simulink model "gmp_pmsm_sensored_nonlinear_sil_mdl_2022b"  (R2022b)
settings: Solver=VariableStepAuto  StartTime=0.0  StopTime=10  RelTol=1e-3
model workspace (MAT data in the model file):
  B = 0
  BW_i = 800
  Flux_t = 0.05895
  IQ24 = Simulink.NumericType
  IQ24.DataTypeMode = 'Fixed-point: binary point scaling'
  IQ24.SignednessBool = 1
  IQ24.WordLength = 32
  IQ24.FixedExponent = -16
  IQ24.SlopeAdjustmentFactor = 1
  IQ24.Bias = 0
  IQ24.DataTypeOverride = 'Inherit'
  IQ24.IsAlias = 0
  IQ24.DataScope = 'Auto'
  J = 0.018
  K_d = 3.72061852168
  K_m = 0.128242020589
  K_u = 0.00236407598332
  Ki_id = 0.001
  Ki_iq = 1
  Ki_n = 25225.1136556
  Kp_id = 1e-05
  Kp_iq = 5e-05
  Kp_n = 12.6125568278
  Ld_t = 0.00303
  Lq_t = 0.02019
  Max_p = 0.006000830667
  P = 2
  RLS_ini_a = 1000000
  Rd_mos = 0.01
  Rs = 0.1215
  Rv = 6.4
  T_final = 0
  T_initial = 0
  Tes = [4 7 10 7 4]
  Tf_t = 0.1
  Tm = 0
  Udq_limit = 550
  Var = 0
  Vce0 = 0
  Vd0 = 0
  Vdc = 80
  button = 1
  im_limit = 40
  mean_prd = 10
  position_init = 0.2
  r_ce = 1e-08
  r_d = 1e-08
  sample_prd = 100
  step_time = 0.2
  ts = 6.25e-05
  wc = 3500
libraries: peripheral_utilities x12, spsSeriesRLCBranchLib x6, spsVoltageMeasurementLib x2, gmp_sil_core_pack x1, spsPermanentMagnetSynchronousMachineLib x1, spsdq0toabcLib x1, spsFourierLib x1, spsControlledVoltageSourceLib x1, spspowerguiLib x1
(part 1 of 2)
settings Model: SimulationMode=accelerator  Creator=javnson  LastModifiedBy=Lin Minyi

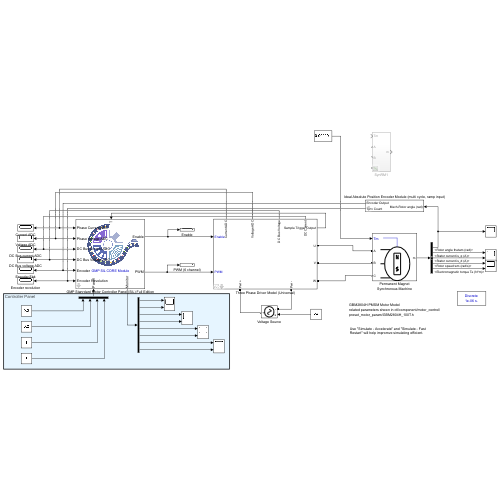
[thumbnail: Simulink's stored preview of the top-level diagram]
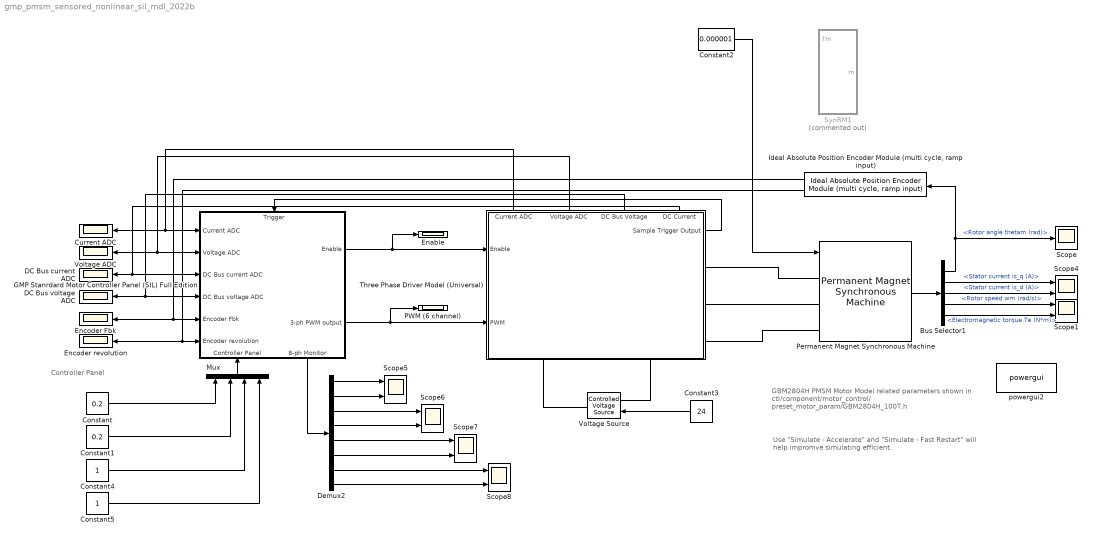
== system gmp_pmsm_sensored_nonlinear_sil_mdl_2022b ==
  note: Use "Simulate - Accelerate" and "Simulate - Fast Restart" will help impromve simulating efficient.
  note: Controller Panel
  note: GBM2804H PMSM Motor Model
      | related parameters shown in ctl/component/motor_control/
      | preset_motor_param/GBM2804H_100T.h
  Bus Selector1 : BusSelector  OutputSignals=Rotor angle thetam (rad),Stator current is_q (A),Stator current is_d (A),Rotor speed wm (rad/s),Electromagnetic torque Te (N*m)
  Constant : Constant  Value=0.2
  Constant1 : Constant  Value=0.2
  Constant2 : Constant  Value=0.000001
  Constant3 : Constant  Value=24
  Constant4 : Constant
  Constant5 : Constant
  Current ADC : Scope
  DC Bus current ADC : Scope
  DC Bus voltage ADC : Scope
  Demux2 : Demux  Outputs=8
  Enable : Scope
  Encoder Fbk : Scope
  Encoder revolution : Scope
  GMP Stanrdard Motor Controller Panel (SIL) Full Edition : Subsystem  mask(GMP SIL Core for single Motor Controller (full edition)){}
      mask help: This is GMP Motor Simulator port.
      settings: PortSchema="{\"entries\":[{\"content\":{\"sides\":[{\"content\":{\"connectorIds\":[\"In1\",\"In2\",\"In3\",\"In4\",\"In5\",\"In6\"]},\"type\":\"ConnectorPlacement.EquallySpacedRectSide\",\"uuid\":\"45c67bc9-9540-469a-a4ac-1e12eb9acca3\"},{\"content\":{\"connectorIds\":[\"Out1\",\"Out2\"],\"side\":\"RIGHT\"},\"type\":\"ConnectorPlacement.EquallySpacedRectSide\",\"uuid\":\"a17116b4-0460-48ab-8ada-a785da6c5e29\"},{\"content\":{\"connectorIds\":[\"In7\"],\"side\":\"TOP\"},\"type\":\"ConnectorPlacement.EquallySpacedRectSide\",\"uuid\":\"15623697-512e-4e4d-ab51-f53c2346fadb\"},{\"content\":{\"connectorIds\":[\"In8\",\"Out3\"],\"side\":\"BOTTOM\"},\"type\":\"ConnectorPlacement.EquallySpacedRectSide\",\"uuid\":\"47f7968c-22c1-4f3d-97d9-242e9dbf8d30\"}]},\"type\":\"ConnectorPlacement.EquallySpacedConnector\",\"uuid\":\"f369880c-e675-4c1f-982e-a4befb03f503\"}],\"packageUris\":[\"http://schema.mathworks.com/mf0/Connector/R2020b\"],\"version\":\"1.0\"}"
      mask DialogControl ParameterGroupVar Prompt: 参数
      mask Display:
      | image(append(fileparts(which('gmp_simulink_utilities.slx')),'\icon\GMP_Core.png'));
      | color('blue');
      | %text(0.3,0.3,'GMP SIL CORE Module','horizontalAlignment','left','verticalAlignment','bottom');
      | disp('\n\n\n\n\n\n\n\nGMP SIL CORE Module');
      | %text(0,0,'y=a*x^2+b','horizontalAlignment','middle', 'verticalAlignment','bottom');
      | 
      | 
      | module_pos = get_param(gcb, 'Position');
      | width = module_pos(3) - module_pos(1);
      | %rectangle('Position',[module_pos(1),module_pos(2),module_pos(3),module_pos(4)],'FaceColor','r');
      | 
      | color('Black');
      | 
      | port_label('output', 1, 'Enable');
      | port_label('output', 2, 'PWM');
      | port_label('output', 3, 'Monitor');
      | 
      | port_label('input', 1, 'Phase Current ADC');
      | port_label('input', 2, 'Phase Voltage ADC');
      | port_label('input', 3, 'DC Bus Current ADC');
      | port_label('input', 4, 'DC Bus Voltage ADC');
      | port_label('input', 5, 'Encoder');
      | port_label('input', 6, 'Encoder Revolution');
      | port_label('input', 7, 'T');
      | port_label('input', 8, 'Panel');
  "Ideal Absolute Position Encoder Module (multi cycle, ramp input)" : peripheral_utilities/Ideal Absolute Position Encoder Module (multi cycle, ramp input)  ENCODER_BIT=14
      settings: SourceProductName=GMP Utilities Library
  Mux : Mux
  PWM (6 channel) : Scope
  Permanent Magnet Synchronous Machine : spsPermanentMagnetSynchronousMachineLib/Permanent Magnet Synchronous Machine  NbPhases=3  FluxDistribution=Sinusoidal  RotorType=Round  MechanicalLoad=Torque Tm  PresetModel=No  ShowDetailedParameters=on  MeasurementBus=off  Resistance=4.7  Inductance=8.5e-3  dqInductances=[8.5e-3,8.5e-3]  La=0.96e-3  MachineConstant=Voltage Constant (V_peak L-L / krpm)  Flux=0.0038197  VoltageCst=1000/206.2  TorqueCst=0.040106  Flat=120  Mechanical=[497e-9 1755e-9 7 0]  PolePairs=4  InitialConditions=[0, 0, 0, 0]  InitialConditions5ph=[0 0 0 0 0 0]  RefAngle=Aligned with phase A axis (original Park)  IterativeDiscreteModel=Trapezoidal non iterative  TsBlock=-1  TsPowergui=0
  Scope : Scope
  Scope{1,4..8} (6 alike) : Scope  NumInputPorts=2
  SynRM1 : Subsystem  Commented=on
  Three Phase Driver Model (Universal) : Subsystem  AncestorBlock=peripheral_utilities/Three Phase Driver Model (Universal)  mask{fswitch=8000, CMP_MAX=6000, Deadband_Upper=48, Deadband_Lower=48, Deadband_us=1, phase_shift=0, R_mosfet_on=0.1, Lon=0, Rd=0.01, Vf=0.3, Rs=1e5, Cs=inf, Rsap=0.005, ADC_GAIN=20, ADC_BIT=12, ADC_REFERENCE=3.3, ADC_BIAS=1.65, ADC_INIT=0, VOLTAGE_ADC_GAIN=0.04049127, VOLTAGE_ADC_BIT=12, VOLTAGE_ADC_REFERENCE=3.3, VOLTAGE_ADC_VOLTAGE=0, VOLTAGE_ADC_INIT=0, VOLTAGE_ADC_CUT_FREQ=1143.4, DCBUS_ADC_GAIN=0.04049127, DCBUS_ADC_BIT=12, DCBUS_ADC_REFERENCE=3.3, DCBUS_ADC_BIAS=0, DCBUS_ADC_INIT=0, DCBUS_CURRENT_ADC_GAIN=1, DCBUS_CURRENT_ADC_BIT=12, DCBUS_CURRENT_ADC_REFERENCE=20, DCBUS_CURRENT_ADC_BIAS=0, DCBUS_CURRENT_ADC_INIT=0}
      mask prompts: DCBUS_CURRENT_ADC_GAIN "DCBUS_ADC_GAIN:"; DCBUS_CURRENT_ADC_BIT "DCBUS_ADC_BIT:"; DCBUS_CURRENT_ADC_REFERENCE "DCBUS_ADC_REFERENCE:"; DCBUS_CURRENT_ADC_BIAS "DCBUS_ADC_BIAS:"; DCBUS_CURRENT_ADC_INIT "DCBUS_ADC_INIT:"
      mask init:
      | calculate_deadband(gcb, 'Deadband_Upper', 'Deadband_Lower',	'CMP_MAX', 'fswitch', 'Deadband_us');
      settings: PortSchema="{\"entries\":[{\"content\":{\"sides\":[{\"content\":{\"connectorIds\":[\"In1\",\"In2\"]},\"type\":\"ConnectorPlacement.EquallySpacedRectSide\",\"uuid\":\"3f4c86ad-0582-4f47-8583-a8af9a7f9adc\"},{\"content\":{\"connectorIds\":[\"Out1\",\"RConn1\",\"RConn2\",\"RConn3\"],\"side\":\"RIGHT\"},\"type\":\"ConnectorPlacement.EquallySpacedRectSide\",\"uuid\":\"ae91f325-3014-4188-9063-296f4d5623fa\"},{\"content\":{\"connectorIds\":[\"Out2\",\"Out3\",\"Out4\",\"Out5\"],\"side\":\"TOP\"},\"type\":\"ConnectorPlacement.EquallySpacedRectSide\",\"uuid\":\"5f2edb36-6849-4a72-b7bd-4d267f120ce4\"},{\"content\":{\"connectorIds\":[\"RConn4\",\"RConn5\"],\"side\":\"BOTTOM\"},\"type\":\"ConnectorPlacement.EquallySpacedRectSide\",\"uuid\":\"79a111ed-6591-4ced-9242-67ea1247c580\"}]},\"type\":\"ConnectorPlacement.EquallySpacedConnector\",\"uuid\":\"8c66eb8e-d25c-472f-a4a5-d1759225ba1c\"}],\"packageUris\":[\"http://schema.mathworks.com/mf0/Connector/R2020b\"],\"version\":\"1.0\"}"
      mask Callback fswitch: calculate_deadband(gcb, 'Deadband_Upper', 'Deadband_Lower',	'CMP_MAX', 'fswitch', 'Deadband_us');
      mask Callback CMP_MAX: calculate_deadband(gcb, 'Deadband_Upper', 'Deadband_Lower',	'CMP_MAX', 'fswitch', 'Deadband_us');
      mask Callback Deadband_Upper: calculate_deadband(gcb, 'Deadband_Upper', 'Deadband_Lower',	'CMP_MAX', 'fswitch', 'Deadband_us');
      mask Callback Deadband_Lower: calculate_deadband(gcb, 'Deadband_Upper', 'Deadband_Lower',	'CMP_MAX', 'fswitch', 'Deadband_us');
      mask DialogControl DescGroupVar Prompt: Three Phases Bridge Peripheral(3-shunt sample)
      mask DialogControl Control21 Prompt: GMP CTL Simulink Utilities: virtual peripherals
      mask DialogControl DescTextVar Prompt: This module provide a ideal 3-phases bridge peripheral.
      mask DialogControl Container4 Prompt: PWM config
      mask DialogControl ParameterGroupVar Prompt: PWM parameters
      mask DialogControl Control2 Prompt: PWM Frequency (Hz):
      mask DialogControl Control4 Prompt: Full Scale PWM Compare value:
      mask DialogControl Control5 Prompt: Deadband Range Set (CMP Value):
      mask DialogControl Control6 Prompt: Deadband time: DEADBAND_CMP/2/CMP_MAX/fswitch
      mask DialogControl Control22 Prompt: Calculated Deadband, us
      mask DialogControl Control20 Prompt: Initial Phase shift:
      mask DialogControl Container5 Prompt: MOSFET config
      mask DialogControl Container7 Prompt: MOSFET parameters
      mask DialogControl Control7 Prompt: Rds(on), unit Ohm
      mask DialogControl Control8 Prompt: Internal diode inducctance, unit H
      mask DialogControl Control9 Prompt: Internal diode resistance Rd, unit Ohm
      mask DialogControl Control10 Prompt: Internal diode forward voltage Vf, unit V
      mask DialogControl Control11 Prompt: Snubber resistance Rs, unit ohm
      mask DialogControl Control12 Prompt: Snubber Capacitance Cs, unit F
      mask DialogControl Container6 Prompt: 3-shunt Current Sample
      mask DialogControl Control13 Prompt: ADC(p.u.) = (real_voltage * ADC_GAIN + ADC_BIAS)/ADC_REFERENCE
      mask DialogControl Control15 Prompt: Shunt Smaple Res, unit Ohm
      mask DialogControl Control14 Prompt: ADC Voltage Gain (Scale Factor):
      mask DialogControl Control16 Prompt: ADC resolution:
      mask DialogControl Control17 Prompt: ADC reference Voltage(V)
      mask DialogControl Control18 Prompt: ADC Bias Voltage(V)
      mask DialogControl Control19 Prompt: ADC Initial Voltage Output (V):
      mask DialogControl Container9 Prompt: 3-shunt Voltage Sample
      mask DialogControl Control34 Prompt: ADC Voltage Gain (Scale Factor):
      mask DialogControl Control23 Prompt: ADC resolution:
      mask DialogControl Control24 Prompt: ADC reference voltage (V), when VOLTAGE_ADC_GAIN = 1, ADC_REF = ADC Full scale
      mask DialogControl Control25 Prompt: ADC Bias Voltage (V):
      mask DialogControl Control26 Prompt: ADC Initial Voltage Output (V):
      mask DialogControl Control27 Prompt: Voltage Filter cut frequency (Hz):
      mask DialogControl Control28 Prompt: Generally, this value less than switch frequency / 10, greater than motor normal frequency * 3
      mask DialogControl Container10 Prompt: DC Bus Voltage Sample
      mask DialogControl Control29 Prompt: ADC Voltage Gain (Scale Factor):
      mask DialogControl Control30 Prompt: ADC resolution:
      mask DialogControl Control32 Prompt: ADC reference voltage (V), when VOLTAGE_ADC_GAIN = 1, ADC_REF = ADC Full scale
      mask DialogControl Control31 Prompt: ADC Bias Voltage (V):
      mask DialogControl Control33 Prompt: ADC Initial Voltage Output (V):
      mask DialogControl Container13 Prompt: DC Bus Current Sample
      mask DialogControl Control29_copy_copy Prompt: ADC Current Gain (Scale Factor):
      mask DialogControl Control30_copy_copy Prompt: ADC resolution:
      mask DialogControl Control32_copy_copy Prompt: ADC reference current (A), when VOLTAGE_ADC_GAIN = 1, ADC_REF = ADC Full scale
      mask DialogControl Control31_copy Prompt: ADC Bias Current (A):
      mask DialogControl Control33_copy Prompt: ADC Initial Current Output (A):
  Voltage ADC : Scope
  Voltage Source : spsControlledVoltageSourceLib/Controlled Voltage Source  Initialize=on  Source_Type=AC  Amplitude=0  Phase=0  Frequency=0  Measurements=None
  powergui2 : spspowerguiLib/powergui  Priority=1  SimulationMode=Discrete  SampleTime=1e-6  frequency=60  Iterations=50  frequencyindice=0  Pbase=100e6  ErrMax=1e-4  UnitsV=kV  UnitsW=MW  buscounter=0  FunctionMessages=off  echomessages=off  EnableUseOfTLC=off  CurrentSourceSwitches=off  DisableSnubberDevices=off  DisableRonSwitches=off  DisableVfSwitches=off  DisplayEquations=off  AutomaticDiscreteSolvers=off  SolverType=Tustin/Backward Euler (TBE)  Interpol=off  ExternalGateDelay=off  methode=off  Ts=100  x0status=blocks  SPID=on  SwTol=0  HookPort=off  NonlinearTolerance=1e-4  nMaxIteration=100  ContinueOnMaxIteration=off  RestoreLinks=warning  ResistiveCurrentMeasurement=off  Frange=[0:2:500]  Ylog=off  Xlog=on  ShowGrid=off  save=off  variable=ZData  structure=0  ZoomFFT=off  StartTime=0.0  cycles=1  DisplayStyle=1  fundamental=60  FreqAxis=off  MaxFrequency=1000  frequencyindicesteady=1  RmsSteady=1  display=off
  wires:
  GMP Stanrdard Motor Controller Panel (SIL) Full Edition/1(Enable) -> Three Phase Driver Model (Universal)/1(Enable), Enable/1
  GMP Stanrdard Motor Controller Panel (SIL) Full Edition/2(3-ph PWM output) -> PWM (6 channel)/1, Three Phase Driver Model (Universal)/2(PWM)
  Constant2/1 -> Permanent Magnet Synchronous Machine/1
  Three Phase Driver Model (Universal)/1(Sample Trigger Output) -> GMP Stanrdard Motor Controller Panel (SIL) Full Edition/7(Trigger)
  Three Phase Driver Model (Universal)/2(Current ADC) -> GMP Stanrdard Motor Controller Panel (SIL) Full Edition/1(Current ADC), Current ADC/1
  Three Phase Driver Model (Universal)/3(Voltage ADC) -> GMP Stanrdard Motor Controller Panel (SIL) Full Edition/2(Voltage ADC), Voltage ADC/1
  Three Phase Driver Model (Universal)/4(DC Bus Voltage) -> DC Bus voltage ADC/1, GMP Stanrdard Motor Controller Panel (SIL) Full Edition/4(DC Bus voltage ADC)
  Permanent Magnet Synchronous Machine/1 -> Bus Selector1/1
  Bus Selector1/1 -> "Ideal Absolute Position Encoder Module (multi cycle, ramp input)"/1, Scope/1  "<Rotor angle thetam (rad)>"
  "Ideal Absolute Position Encoder Module (multi cycle, ramp input)"/1 -> Encoder Fbk/1, GMP Stanrdard Motor Controller Panel (SIL) Full Edition/5(Encoder Fbk)
  Bus Selector1/3 -> Scope4/2  "<Stator current is_d (A)>"
  Bus Selector1/2 -> Scope4/1  "<Stator current is_q (A)>"
  Constant3/1 -> Voltage Source/1
  Demux2/4 -> Scope6/2
  Demux2/3 -> Scope6/1
  Demux2/2 -> Scope5/2
  Demux2/1 -> Scope5/1
  GMP Stanrdard Motor Controller Panel (SIL) Full Edition/3(8-ph Monitor) -> Demux2/1
  Bus Selector1/4 -> Scope1/1  "<Rotor speed wm (rad/s)>"
  Bus Selector1/5 -> Scope1/2  "<Electromagnetic torque Te (N*m)>"
  "Ideal Absolute Position Encoder Module (multi cycle, ramp input)"/2 -> Encoder revolution/1, GMP Stanrdard Motor Controller Panel (SIL) Full Edition/6(Encoder revolution)
  Mux/1 -> GMP Stanrdard Motor Controller Panel (SIL) Full Edition/8(Controller Panel)
  Constant/1 -> Mux/1
  Constant1/1 -> Mux/2
  Constant4/1 -> Mux/3
  Constant5/1 -> Mux/4
  Demux2/5 -> Scope7/1
  Demux2/6 -> Scope7/2
  Demux2/7 -> Scope8/1
  Demux2/8 -> Scope8/2
  Three Phase Driver Model (Universal)/5(DC Current) -> DC Bus current ADC/1, GMP Stanrdard Motor Controller Panel (SIL) Full Edition/3(DC Bus current ADC)
  connections:
  Permanent Magnet Synchronous Machine/LConn2 -- Three Phase Driver Model (Universal)/RConn2
  Permanent Magnet Synchronous Machine/LConn3 -- Three Phase Driver Model (Universal)/RConn3
  Permanent Magnet Synchronous Machine/LConn1 -- Three Phase Driver Model (Universal)/RConn1
  Three Phase Driver Model (Universal)/RConn5 -- Voltage Source/LConn1
  Three Phase Driver Model (Universal)/RConn4 -- Voltage Source/RConn1

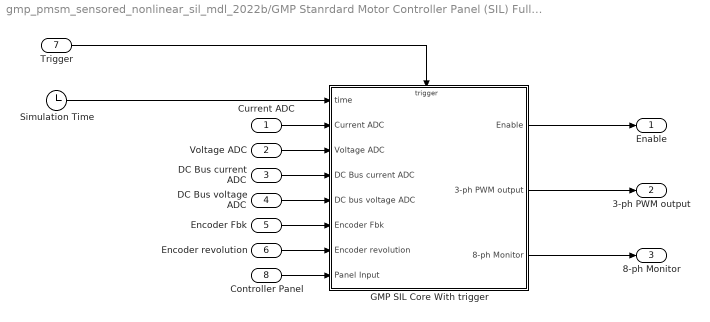
== system gmp_pmsm_sensored_nonlinear_sil_mdl_2022b/GMP Stanrdard Motor Controller Panel (SIL) Full Edition ==
  Current ADC : Inport
  Voltage ADC : Inport  Port=2
  DC Bus current ADC : Inport  Port=3
  DC Bus voltage ADC : Inport  Port=4
  Encoder Fbk : Inport  Port=5
  Encoder revolution : Inport  Port=6
  Trigger : Inport  Port=7
  Controller Panel : Inport  Port=8
  GMP SIL Core With trigger : Subsystem
  Simulation Time : Clock
  Enable : Outport
  3-ph PWM output : Outport  Port=2
  8-ph Monitor : Outport  Port=3
  wires:
  Encoder Fbk/1 -> GMP SIL Core With trigger/6(Encoder Fbk)
  Encoder revolution/1 -> GMP SIL Core With trigger/7(Encoder revolution)
  GMP SIL Core With trigger/2(3-ph PWM output) -> 3-ph PWM output/1
  Simulation Time/1 -> GMP SIL Core With trigger/1(time)
  GMP SIL Core With trigger/1(Enable) -> Enable/1
  Voltage ADC/1 -> GMP SIL Core With trigger/3(Voltage ADC)
  Current ADC/1 -> GMP SIL Core With trigger/2(Current ADC)
  GMP SIL Core With trigger/3(8-ph Monitor) -> 8-ph Monitor/1
  DC Bus current ADC/1 -> GMP SIL Core With trigger/4(DC Bus current ADC)
  Trigger/1 -> GMP SIL Core With trigger/Trigger
  DC Bus voltage ADC/1 -> GMP SIL Core With trigger/5(DC bus voltage ADC)
  Controller Panel/1 -> GMP SIL Core With trigger/8(Panel Input)

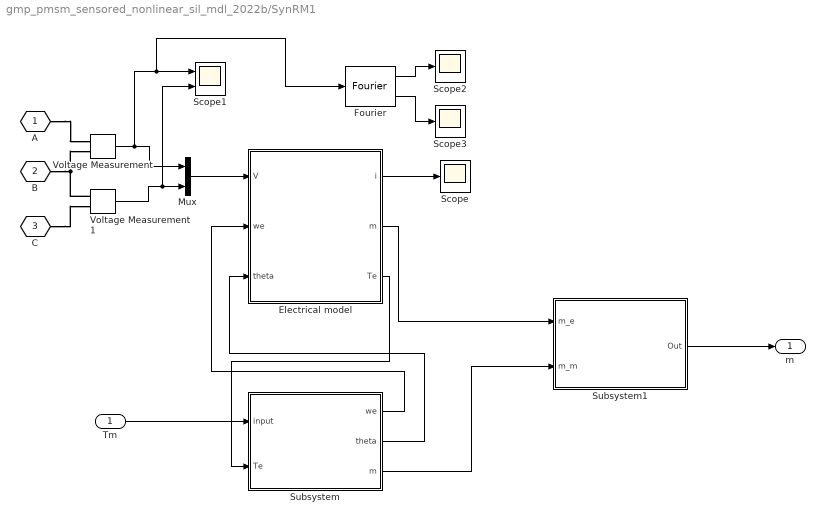
== system gmp_pmsm_sensored_nonlinear_sil_mdl_2022b/SynRM1 ==
  Tm : Inport
  Electrical model : Subsystem
  Fourier : spsFourierLib/Fourier  Freq=100  n=1  InInit=[0, 0]  Ts=0
  Mux : Mux  Inputs=2
  Scope : Scope
  Scope1 : Scope  NumInputPorts=2
  Scope2 : Scope
  Scope3 : Scope
  Subsystem : Subsystem
  Subsystem1 : Subsystem
  Voltage Measurement : spsVoltageMeasurementLib/Voltage Measurement  PhasorSimulation=off  OutputType=Complex  PSBequivalent=0
  Voltage Measurement1 : spsVoltageMeasurementLib/Voltage Measurement  PhasorSimulation=off  OutputType=Complex  PSBequivalent=0
  A : PMIOPort  Side=Left
  B : PMIOPort  Port=2  Side=Left
  C : PMIOPort  Port=3  Side=Left
  m : Outport  VectorParamsAs1DForOutWhenUnconnected=off
  wires:
  Subsystem/3(m) -> Subsystem1/2(m_m)
  Subsystem/1(we) -> Electrical model/2(we)
  Mux/1 -> Electrical model/1(V)
  Subsystem/2(theta) -> Electrical model/3(theta)
  Electrical model/3(Te) -> Subsystem/2(Te)
  Subsystem1/1(Out) -> m/1
  Electrical model/1(i) -> Scope/1
  Electrical model/2(m) -> Subsystem1/1(m_e)
  Tm/1 -> Subsystem/1(input)
  Voltage Measurement/1 -> Fourier/1, Scope1/1, Mux/1
  Voltage Measurement1/1 -> Scope1/2, Mux/2
  Fourier/1 -> Scope2/1
  Fourier/2 -> Scope3/1
  connections:
  C/RConn1 -- Voltage Measurement1/LConn2
  A/RConn1 -- Voltage Measurement/LConn1
  B/RConn1 -- Voltage Measurement1/LConn1 -- Voltage Measurement/LConn2

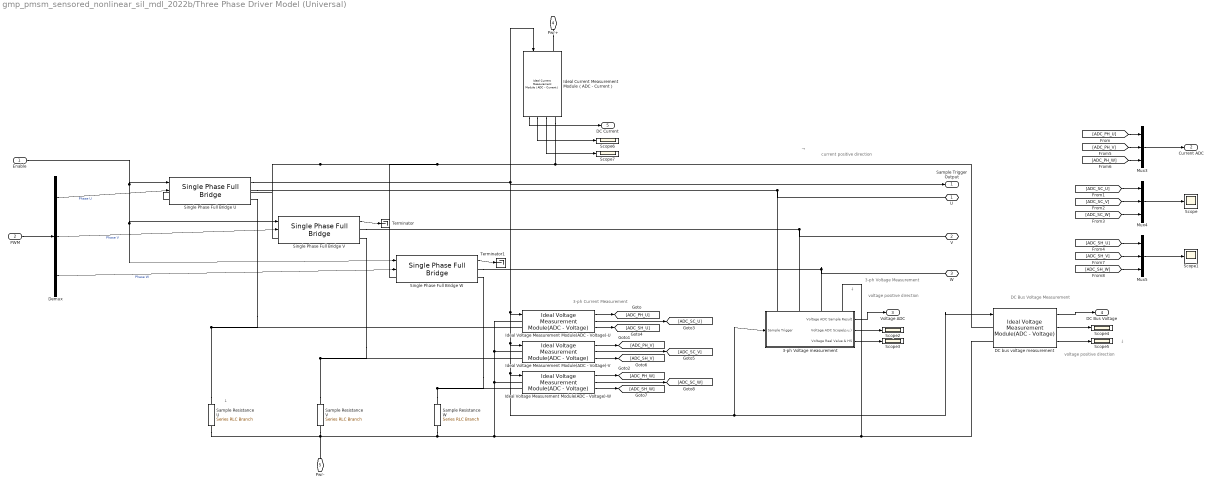
== system gmp_pmsm_sensored_nonlinear_sil_mdl_2022b/Three Phase Driver Model (Universal) ==
  note: 3-ph Current Measurement
  note: →
  note: current positive direction
  note: ↓
  note: voltage positive direction
  note: ↓
  note: 3-ph Voltage Measurement
  note: DC Bus Voltage Measurement
  note: ↓
  note: voltage positive direction
  Enable : Inport
  PWM : Inport  Port=2
  3-ph Voltage measurement : Subsystem  AncestorBlock=peripheral_utilities/Three Phases Voltage (ph-gnd) Measurement with Filter  mask{ADC_GAIN=VOLTAGE_ADC_GAIN, ADC_BIT=VOLTAGE_ADC_BIT, ADC_REFERENCE=VOLTAGE_ADC_REFERENCE, ADC_BIAS=VOLTAGE_ADC_VOLTAGE, ADC_INIT=VOLTAGE_ADC_INIT, cut_frequency=VOLTAGE_ADC_CUT_FREQ}
      settings: PortSchema="{\"entries\":[{\"content\":{\"sides\":[{\"content\":{\"connectorIds\":[\"In1\"]},\"type\":\"ConnectorPlacement.EquallySpacedRectSide\",\"uuid\":\"ae4f4612-c092-4fa0-8a43-5c9e823110e3\"},{\"content\":{\"connectorIds\":[\"Out1\",\"Out2\",\"Out3\"],\"side\":\"RIGHT\"},\"type\":\"ConnectorPlacement.EquallySpacedRectSide\",\"uuid\":\"6db15ef0-d33a-4775-b4e6-14a566796673\"},{\"content\":{\"connectorIds\":[\"LConn1\",\"LConn2\",\"LConn3\",\"LConn4\"],\"side\":\"TOP\"},\"type\":\"ConnectorPlacement.EquallySpacedRectSide\",\"uuid\":\"cfddd664-59f3-497b-b33e-fe832fe7a7bd\"}]},\"type\":\"ConnectorPlacement.EquallySpacedConnector\",\"uuid\":\"5bacf0ad-0c4a-4f47-a242-d8a476ab7f52\"}],\"packageUris\":[\"http://schema.mathworks.com/mf0/Connector/R2020b\"],\"version\":\"1.0\"}"
      mask DialogControl DescGroupVar Prompt: 3 phases Voltage Sample ADC Model
      mask DialogControl Control10 Prompt: GMP CTL Simulink Utilities: virtual peripherals
      mask DialogControl DescTextVar Prompt: This is a ideal Voltage Measurement Module.
      mask DialogControl Control2 Prompt: ADC(p.u.) = (real_voltage * ADC_GAIN + ADC_BIAS)/ADC_REFERENCE
      mask DialogControl ParameterGroupVar Prompt: parameters:
      mask DialogControl Control3 Prompt: ADC Voltage Gain (Scale Factor):
      mask DialogControl Control4 Prompt: ADC resolution:
      mask DialogControl Control5 Prompt: ADC reference Voltage (V), when ADC_GAIN=1, ADC_REF = ADC full scale
      mask DialogControl Control6 Prompt: ADC Bias Voltage(V)
      mask DialogControl Control7 Prompt: ADC Initial Voltage Output (V):
      mask DialogControl Control8 Prompt: Voltage Filter cut frequency (Hz):
      mask DialogControl Control9 Prompt: Generally, this value less than switch frequency / 10, greater than motor normal frequency * 3
  DC bus voltage measurement : peripheral_utilities/Ideal Voltage Measurement Module(ADC - Voltage)  ADC_GAIN=DCBUS_ADC_GAIN  ADC_BIT=DCBUS_ADC_BIT  ADC_REFERENCE=DCBUS_ADC_REFERENCE  ADC_BIAS=DCBUS_ADC_BIAS  ADC_INIT=DCBUS_ADC_INIT
      settings: SourceProductName=GMP Utilities Library
  Demux : Demux  Outputs=3
  Ideal Current Measurement Module（ADC - Current） : peripheral_utilities/Ideal Current Measurement Module（ADC - Current）  ADC_GAIN=DCBUS_CURRENT_ADC_GAIN  ADC_BIT=DCBUS_CURRENT_ADC_BIT  ADC_REFERENCE=DCBUS_CURRENT_ADC_REFERENCE  ADC_BIAS=DCBUS_CURRENT_ADC_BIAS  ADC_INIT=DCBUS_CURRENT_ADC_INIT
      settings: SourceProductName=GMP Utilities Library
  Ideal Voltage Measurement Module(ADC - Voltage)-U : peripheral_utilities/Ideal Voltage Measurement Module(ADC - Voltage)  ADC_GAIN=ADC_GAIN  ADC_BIT=ADC_BIT  ADC_REFERENCE=ADC_REFERENCE  ADC_BIAS=ADC_BIAS  ADC_INIT=ADC_INIT
      settings: SourceProductName=GMP Utilities Library
  Ideal Voltage Measurement Module(ADC - Voltage)-V : peripheral_utilities/Ideal Voltage Measurement Module(ADC - Voltage)  ADC_GAIN=ADC_GAIN  ADC_BIT=ADC_BIT  ADC_REFERENCE=ADC_REFERENCE  ADC_BIAS=ADC_BIAS  ADC_INIT=ADC_INIT
      settings: SourceProductName=GMP Utilities Library
  Ideal Voltage Measurement Module(ADC - Voltage)-W : peripheral_utilities/Ideal Voltage Measurement Module(ADC - Voltage)  ADC_GAIN=ADC_GAIN  ADC_BIT=ADC_BIT  ADC_REFERENCE=ADC_REFERENCE  ADC_BIAS=ADC_BIAS  ADC_INIT=ADC_INIT
      settings: SourceProductName=GMP Utilities Library
  Mux3 : Mux  Inputs=3
  Mux4 : Mux  Inputs=3
  Mux5 : Mux  Inputs=3
  Sample Resistance U : spsSeriesRLCBranchLib/Series RLC Branch  LConnTagsString=__new0  RConnTagsString=__new0  BranchType=R  Resistance=Rsap  Inductance=1e-3  SetiL0=off  InitialCurrent=0  Capacitance=1e-6  Setx0=off  InitialVoltage=0  Measurements=None
  Sample Resistance V : spsSeriesRLCBranchLib/Series RLC Branch  LConnTagsString=__new0  RConnTagsString=__new0  BranchType=R  Resistance=Rsap  Inductance=1e-3  SetiL0=off  InitialCurrent=0  Capacitance=1e-6  Setx0=off  InitialVoltage=0  Measurements=None
  Sample Resistance W : spsSeriesRLCBranchLib/Series RLC Branch  LConnTagsString=__new0  RConnTagsString=__new0  BranchType=R  Resistance=Rsap  Inductance=1e-3  SetiL0=off  InitialCurrent=0  Capacitance=1e-6  Setx0=off  InitialVoltage=0  Measurements=None
  Scope{,1..7} (8 alike) : Scope
  Single Phase Full Bridge U : peripheral_utilities/Single Phase Full Bridge  fswitch=fswitch  CMP_MAX=CMP_MAX  Deadband_Upper=Deadband_Upper  Deadband_Lower=Deadband_Lower  Deadband_us=NaN  phase_shift=phase_shift  R_mosfet_on=R_mosfet_on  Lon=Lon  Rd=Rd  Vf=Vf  Rs=Rs  Cs=Cs
      settings: SourceProductName=GMP Utilities Library
  Single Phase Full Bridge V : peripheral_utilities/Single Phase Full Bridge  fswitch=fswitch  CMP_MAX=CMP_MAX  Deadband_Upper=Deadband_Upper  Deadband_Lower=Deadband_Lower  Deadband_us=NaN  phase_shift=phase_shift  R_mosfet_on=R_mosfet_on  Lon=Lon  Rd=Rd  Vf=Vf  Rs=Rs  Cs=Cs
      settings: SourceProductName=GMP Utilities Library
  Single Phase Full Bridge W : peripheral_utilities/Single Phase Full Bridge  fswitch=fswitch  CMP_MAX=CMP_MAX  Deadband_Upper=Deadband_Upper  Deadband_Lower=Deadband_Lower  Deadband_us=NaN  phase_shift=phase_shift  R_mosfet_on=R_mosfet_on  Lon=Lon  Rd=Rd  Vf=Vf  Rs=Rs  Cs=Cs
      settings: SourceProductName=GMP Utilities Library
  Terminator : Terminator
  Terminator1 : Terminator
  U : PMIOPort  Side=Right
  V : PMIOPort  Port=2  Side=Right
  W : PMIOPort  Port=3  Side=Right
  Pwr+ : PMIOPort  Port=4  Side=Right
  Pwr- : PMIOPort  Port=5  Side=Right
  Sample Trigger Output : Outport
  Current ADC : Outport  Port=2
  Voltage ADC : Outport  Port=3
  DC Bus Voltage : Outport  Port=4
  DC Current : Outport  Port=5
  wires:
  Demux/1 -> Single Phase Full Bridge U/2  "Phase U"
  Ideal Voltage Measurement Module(ADC - Voltage)-U/1 -> [ADC_PH_U]
  Single Phase Full Bridge V/1 -> Terminator/1
  Single Phase Full Bridge W/1 -> Terminator1/1
  Ideal Voltage Measurement Module(ADC - Voltage)-U/2 -> [ADC_SC_U]
  Demux/2 -> Single Phase Full Bridge V/2  "Phase V"
  Demux/3 -> Single Phase Full Bridge W/2  "Phase W"
  [ADC_PH_V] -> Mux3/2
  [ADC_SC_V] -> Mux4/2
  Ideal Voltage Measurement Module(ADC - Voltage)-U/3 -> [ADC_SH_U]
  Mux3/1 -> Current ADC/1
  Ideal Voltage Measurement Module(ADC - Voltage)-V/1 -> [ADC_PH_V]
  [ADC_SC_U] -> Mux4/1
  [ADC_SH_W] -> Mux5/3
  Mux5/1 -> Scope1/1
  Ideal Voltage Measurement Module(ADC - Voltage)-W/1 -> [ADC_PH_W]
  [ADC_PH_U] -> Mux3/1
  Enable/1 -> Single Phase Full Bridge V/1, Single Phase Full Bridge W/1, Single Phase Full Bridge U/1
  Mux4/1 -> Scope/1
  Ideal Voltage Measurement Module(ADC - Voltage)-V/3 -> [ADC_SH_V]
  Single Phase Full Bridge U/1 -> Sample Trigger Output/1, Ideal Current Measurement Module（ADC - Current）/1, Ideal Voltage Measurement Module(ADC - Voltage)-V/1, Ideal Voltage Measurement Module(ADC - Voltage)-W/1, DC bus voltage measurement/1, 3-ph Voltage measurement/1(Sample Trigger), Ideal Voltage Measurement Module(ADC - Voltage)-U/1
  [ADC_SH_U] -> Mux5/1
  Ideal Voltage Measurement Module(ADC - Voltage)-V/2 -> [ADC_SC_V]
  Ideal Voltage Measurement Module(ADC - Voltage)-W/3 -> [ADC_SH_W]
  [ADC_PH_W] -> Mux3/3
  [ADC_SC_W] -> Mux4/3
  [ADC_SH_V] -> Mux5/2
  Ideal Voltage Measurement Module(ADC - Voltage)-W/2 -> [ADC_SC_W]
  3-ph Voltage measurement/1(Voltage ADC Sample Result) -> Voltage ADC/1
  3-ph Voltage measurement/2(Voltage ADC Scope(p.u.)) -> Scope2/1
  3-ph Voltage measurement/3(Voltage Real Value & HS) -> Scope3/1
  DC bus voltage measurement/1 -> DC Bus Voltage/1
  DC bus voltage measurement/2 -> Scope4/1
  DC bus voltage measurement/3 -> Scope5/1
  PWM/1 -> Demux/1
  Ideal Current Measurement Module（ADC - Current）/1 -> DC Current/1
  Ideal Current Measurement Module（ADC - Current）/2 -> Scope6/1
  Ideal Current Measurement Module（ADC - Current）/3 -> Scope7/1
  connections:
  Single Phase Full Bridge V/RConn1 -- V/RConn1 -- 3-ph Voltage measurement/LConn2
  Single Phase Full Bridge U/RConn1 -- U/RConn1 -- 3-ph Voltage measurement/LConn1
  Single Phase Full Bridge W/RConn1 -- W/RConn1 -- 3-ph Voltage measurement/LConn3
  Sample Resistance V/LConn1 -- Ideal Voltage Measurement Module(ADC - Voltage)-V/LConn2 -- Single Phase Full Bridge V/RConn2
  Pwr-/RConn1 -- Sample Resistance U/RConn1 -- Sample Resistance V/RConn1 -- Sample Resistance W/RConn1 -- 3-ph Voltage measurement/LConn4 -- DC bus voltage measurement/LConn2 -- Ideal Voltage Measurement Module(ADC - Voltage)-U/LConn1 -- Ideal Voltage Measurement Module(ADC - Voltage)-V/LConn1 -- Ideal Voltage Measurement Module(ADC - Voltage)-W/LConn1
  Sample Resistance W/LConn1 -- Ideal Voltage Measurement Module(ADC - Voltage)-W/LConn2 -- Single Phase Full Bridge W/RConn2
  Sample Resistance U/LConn1 -- Ideal Voltage Measurement Module(ADC - Voltage)-U/LConn2 -- Single Phase Full Bridge U/RConn2
  DC bus voltage measurement/LConn1 -- Ideal Current Measurement Module（ADC - Current）/RConn1 -- Single Phase Full Bridge W/LConn1 -- Single Phase Full Bridge U/LConn1 -- Single Phase Full Bridge V/LConn1
  Pwr+/RConn1 -- Ideal Current Measurement Module（ADC - Current）/LConn1

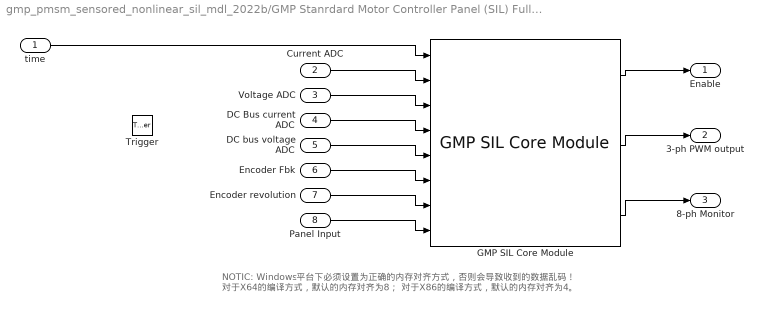
== system gmp_pmsm_sensored_nonlinear_sil_mdl_2022b/GMP Stanrdard Motor Controller Panel (SIL) Full Edition/GMP SIL Core With trigger ==
  note: NOTIC:
      | Windows平台下必须设置为正确的内存对齐方式，否则会导致收到的数据乱码！
      | 对于X64的编译方式，默认的内存对齐为8；
      | 对于X86的编译方式，默认的内存对齐为4。
  time : Inport
  Current ADC : Inport  Port=2
  Voltage ADC : Inport  Port=3
  DC Bus current ADC : Inport  Port=4
  DC bus voltage ADC : Inport  Port=5
  Encoder Fbk : Inport  Port=6
  Encoder revolution : Inport  Port=7
  Panel Input : Inport  Port=8
  Trigger : TriggerPort  VariantControl=(inherit)  PortDimensions=1
  GMP SIL Core Module : gmp_sil_core_pack/GMP SIL Core Module  MaskPackedDataTypes={'double','uint32','uint32','uint32','uint32', 'uint32', 'int32', 'double'}  MaskPackedDataSizes={[1],[3],[3],[1],[1], [1], [1], [4]}  MaskUnpackedDataTypes={'double', 'uint32','double'}  MaskUnpackedDataSizes={[1],[3],[8]}  MaskAlignment=1  MaskHostAddr='127.0.0.1'  MaskMsgTxPort=12300  MaskMsgRxPort=12301  MaskCmdTxPort=12302  MaskCmdRxPort=12303
      settings: SourceProductName=GMP Utilities Library
  Enable : Outport
  3-ph PWM output : Outport  Port=2
  8-ph Monitor : Outport  Port=3
  wires:
  Current ADC/1 -> GMP SIL Core Module/2
  Voltage ADC/1 -> GMP SIL Core Module/3
  DC Bus current ADC/1 -> GMP SIL Core Module/4
  time/1 -> GMP SIL Core Module/1
  GMP SIL Core Module/3 -> 8-ph Monitor/1
  GMP SIL Core Module/2 -> 3-ph PWM output/1
  GMP SIL Core Module/1 -> Enable/1
  Encoder Fbk/1 -> GMP SIL Core Module/6
  Encoder revolution/1 -> GMP SIL Core Module/7
  DC bus voltage ADC/1 -> GMP SIL Core Module/5
  Panel Input/1 -> GMP SIL Core Module/8

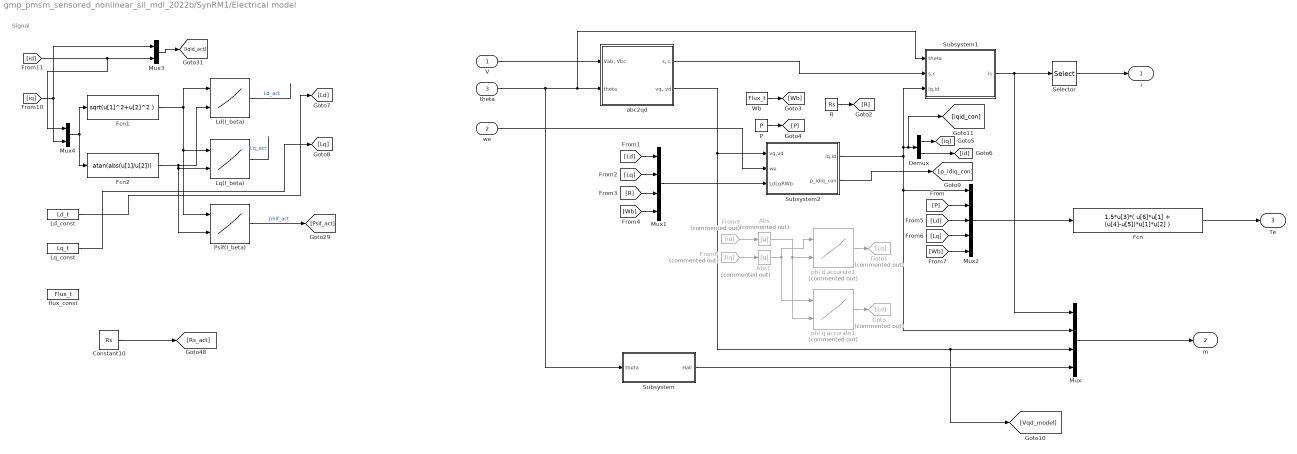
== system gmp_pmsm_sensored_nonlinear_sil_mdl_2022b/SynRM1/Electrical model ==
  note: Signal
  V : Inport
  we : Inport  Port=2
  theta : Inport  Port=3
  Abs : Abs  Commented=on  SaturateOnIntegerOverflow=off
  Abs1 : Abs  Commented=on  SaturateOnIntegerOverflow=off
  Constant10 : Constant  Value=Rs
  Demux : Demux  Outputs=2
  Fcn : Fcn  Expr=1.5*u[3]*( u[6]*u[1] + (u[4]-u[5])*u[1]*u[2] )
  Fcn1 : Fcn  Expr=sqrt(u[1]^2+u[2]^2 )
  Fcn2 : Fcn  Expr=atan(abs(u[1]/u[2]))
  From8 : From  Commented=on  GotoTag=iq
  From9 : From  Commented=on  GotoTag=id
  Goto : Goto  Commented=on  GotoTag=Ld
  Goto1 : Goto  Commented=on  GotoTag=Lq
  Ld(I_beta) : Lookup_n-D  BreakpointsForDimension1=[0,4,8,12,16,20,24,28,32,36,40,44,48,52,56,60,64,68,72,76]  BreakpointsForDimension2=[0,4,8,12,16,20,24,28,32,36,40,44,48,52,56,60,64,68,72,76,80,84,88,90]  Table=[0.0090049,0.0090049,0.0090049,0.0090049,0.0090049,0.0090049,0.0090049,0.0090049,0.0090049,0.0090049,0.0090049,0.0090049,0.0090049,0.0090049,0.0090049,0.0090049,0.0090049,0.0090049,0.0090049,0.0090049,0.0090049,0.0090049,0.0090049,0.0090049;0.0091068,0.0083359,0.0077182,0.0071952,0.0067602,0.0063986,0.0061075,0.0058615,0.0056442,0.0054621,0.0053073,0.0051722,0.0050586,0.0049576,0.0048709,0.0047948,0.0047272,0.0046738,0.0046308,0.0045967,0.00457,0.0045527,0.0045425,0.0045403;0.0093464,0.0079938,0.0070425,0.006355,0.0058504,0.0054685,0.005168,0.004922,0.0047173,0.0045442,0.0044053,0.0042808,0.0041752,0.0040816,0.0040014,0.0039315,0.0038713,0.0038189,0.0037747,0.0037414,0.0037159,0.0036999,0.0036913,0.0036904;0.0094184,0.0086648,0.007532,0.0065799,0.0059032,0.0053778,0.0049522,0.0046235,0.0043749,0.0041848,0.0040338,0.0039102,0.0038062,0.0037163,0.0036343,0.0035659,0.003505,0.0034522,0.0034077,0.003372,0.0033446,0.0033271,0.0033182,0.003317;0.007537,0.0073523,0.0068251,0.0060935,0.0054955,0.0050421,0.0046797,0.0043924,0.0041627,0.0039813,0.0038382,0.003715,0.0036051,0.0035122,0.0034334,0.0033641,0.0033014,0.0032455,0.0031985,0.00316,0.0031309,0.0031118,0.0031022,0.0031011;0.0069136,0.0066119,0.0061429,0.0055601,0.0050595,0.0046689,0.004363,0.0041106,0.0039094,0.0037548,0.0036311,0.0035297,0.003445,0.0033686,0.0032942,0.0032267,0.0031671,0.0031114,0.0030613,0.0030204,0.0029894,0.002969,0.0029587,0.0029574;0.0067888,0.0062678,0.005688,0.0051372,0.0047121,0.0043706,0.0040971,0.0038745,0.0037001,0.0035638,0.0034559,0.0033682,0.0032948,0.0032327,0.0031761,0.0031194,0.0030631,0.0030118,0.0029628,0.0029201,0.0028873,0.0028657,0.002855,0.0028536;0.0064852,0.0059179,0.0053416,0.0048215,0.0044208,0.0041168,0.0038718,0.0036757,0.0035267,0.0034084,0.0033126,0.0032335,0.0031693,0.0031162,0.0030692,0.0030242,0.0029766,0.0029286,0.0028841,0.0028423,0.0028087,0.0027864,0.0027753,0.0027739;0.0061523,0.0056113,0.0050565,0.0045719,0.0041984,0.0039199,0.0036926,0.0035158,0.0033808,0.0032752,0.0031919,0.0031227,0.0030647,0.0030165,0.0029765,0.0029393,0.0029008,0.0028583,0.002817,0.002778,0.0027453,0.0027227,0.0027115,0.0027103;0.0058954,0.0053596,0.0048097,0.0043561,0.0040148,0.0037503,0.0035417,0.0033833,0.0032591,0.0031631,0.0030877,0.0030266,0.0029757,0.0029326,0.0028962,0.0028645,0.0028327,0.0027967,0.0027584,0.0027223,0.002691,0.0026694,0.0026587,0.0026572;0.0056976,0.0051489,0.0045961,0.004167,0.0038525,0.0036066,0.0034122,0.0032677,0.0031545,0.0030661,0.0029972,0.0029426,0.0028976,0.0028598,0.0028271,0.0027991,0.0027724,0.0027421,0.002707,0.0026731,0.0026436,0.0026234,0.0026135,0.0026121;0.0055231,0.0049627,0.0044187,0.0040007,0.0037069,0.0034785,0.0032983,0.0031643,0.0030617,0.0029804,0.0029182,0.0028686,0.0028288,0.0027956,0.0027666,0.0027417,0.0027187,0.0026929,0.0026618,0.0026296,0.0026011,0.0025825,0.0025738,0.0025727;0.0053694,0.0047911,0.0042535,0.0038565,0.0035785,0.0033645,0.0031988,0.0030752,0.0029797,0.0029055,0.0028481,0.0028031,0.002767,0.0027377,0.002713,0.0026907,0.0026708,0.0026487,0.0026213,0.0025909,0.0025632,0.0025454,0.0025381,0.0025373;0.0052237,0.0046319,0.0041064,0.0037302,0.0034662,0.0032628,0.0031101,0.0029956,0.0029078,0.0028387,0.0027859,0.0027449,0.0027117,0.0026861,0.0026645,0.0026452,0.0026275,0.0026087,0.0025847,0.002556,0.0025292,0.0025117,0.0025053,0.0025047;0.0050914,0.0044851,0.003973,0.0036151,0.0033625,0.0031734,0.0030322,0.0029247,0.0028431,0.0027797,0.0027305,0.0026924,0.0026625,0.0026388,0.0026201,0.002604,0.0025886,0.0025725,0.0025511,0.0025243,0.0024983,0.0024809,0.0024746,0.0024742;0.004977,0.004351,0.0038492,0.0035074,0.0032708,0.0030953,0.0029629,0.0028607,0.0027852,0.0027265,0.002681,0.0026455,0.0026177,0.0025961,0.0025796,0.0025663,0.0025528,0.0025391,0.0025203,0.0024953,0.00247,0.0024526,0.002446,0.0024453;0.0048627,0.0042246,0.0037365,0.0034117,0.0031881,0.0030249,0.0028998,0.002804,0.0027327,0.0026783,0.0026359,0.0026029,0.0025771,0.0025573,0.0025427,0.0025312,0.0025199,0.0025084,0.0024918 ...(+761 chars)]  InterpMethod=Akima spline  RndMeth=Simplest
      settings: InputPortMap=u0,u1
  Ld_const : Constant  Value=Ld_t
  Lq(I_beta) : Lookup_n-D  BreakpointsForDimension1=[0,4,8,12,16,20,24,28,32,36,40,44,48,52,56,60,64,68,72,76]  BreakpointsForDimension2=[0,4,8,12,16,20,24,28,32,36,40,44,48,52,56,60,64,68,72,76,80,84,88,90]  Table=[0.027272,0.027272,0.027272,0.027272,0.027272,0.027272,0.027272,0.027272,0.027272,0.027272,0.027272,0.027272,0.027272,0.027272,0.027272,0.027272,0.027272,0.027272,0.027272,0.027272,0.027272,0.027272,0.027272,0.027272;0.027457,0.027451,0.027443,0.027434,0.027425,0.027414,0.027402,0.02739,0.027376,0.027361,0.027345,0.027328,0.027312,0.027294,0.027277,0.02726,0.027243,0.027228,0.027214,0.027202,0.027193,0.027187,0.027183,0.027183;0.027424,0.02742,0.027429,0.027443,0.027463,0.027488,0.027502,0.027506,0.027502,0.027489,0.02747,0.027448,0.02742,0.027389,0.027353,0.027315,0.027274,0.027232,0.02719,0.027153,0.027123,0.027102,0.027091,0.02709;0.024416,0.024514,0.024663,0.024863,0.025117,0.025413,0.025742,0.02607,0.026395,0.026688,0.026936,0.027154,0.027312,0.027386,0.02738,0.027348,0.027301,0.027245,0.027182,0.027117,0.027059,0.027015,0.026992,0.026989;0.02017,0.02027,0.02045,0.020689,0.02099,0.021369,0.02182,0.022355,0.022972,0.023672,0.024447,0.025225,0.025912,0.02649,0.026932,0.027211,0.027268,0.027228,0.027161,0.02708,0.026997,0.026928,0.026888,0.026883;0.017083,0.017167,0.017325,0.017546,0.017836,0.018192,0.018626,0.019145,0.019755,0.020476,0.021306,0.02226,0.023328,0.024442,0.025444,0.02627,0.026871,0.027127,0.027109,0.027029,0.026931,0.026839,0.026782,0.026775;0.014717,0.014798,0.014939,0.015143,0.015413,0.015756,0.016171,0.016667,0.017254,0.017938,0.018741,0.019678,0.02076,0.022,0.023359,0.024679,0.025792,0.026628,0.026978,0.026954,0.026855,0.026746,0.026674,0.026664;0.012887,0.012961,0.013093,0.013279,0.013524,0.013837,0.014221,0.014684,0.015243,0.015903,0.016678,0.017574,0.018624,0.019853,0.021269,0.022834,0.024363,0.025653,0.026571,0.02683,0.026764,0.026648,0.026562,0.026551;0.011447,0.011518,0.01164,0.011811,0.012035,0.012323,0.012674,0.013102,0.013617,0.014233,0.014972,0.015841,0.016854,0.018037,0.019437,0.021055,0.022814,0.024466,0.025829,0.026582,0.026648,0.026543,0.026448,0.026435;0.010299,0.010364,0.010475,0.010633,0.010841,0.011105,0.011431,0.011827,0.012302,0.012874,0.013559,0.01438,0.015359,0.016508,0.01786,0.019466,0.021308,0.023214,0.02491,0.026137,0.026485,0.026425,0.026329,0.026314;0.009364,0.0094217,0.0095231,0.0096707,0.0098639,0.010107,0.010408,0.010777,0.01122,0.011752,0.012391,0.013158,0.014081,0.015193,0.016508,0.018073,0.019924,0.021976,0.023923,0.025531,0.026262,0.02629,0.026204,0.026188;0.0085868,0.0086393,0.0087346,0.0088688,0.0090479,0.0092749,0.0095542,0.0098959,0.010311,0.010809,0.011409,0.01213,0.013,0.014056,0.015331,0.016852,0.018681,0.020793,0.022941,0.024838,0.025951,0.026132,0.02607,0.026056;0.0079329,0.0079796,0.0080672,0.0081916,0.0083583,0.0085706,0.008832,0.0091518,0.0095399,0.010008,0.010572,0.011251,0.012073,0.013074,0.014298,0.015777,0.017569,0.019694,0.021981,0.024103,0.025573,0.025947,0.025924,0.025914;0.0073732,0.0074161,0.0074969,0.0076131,0.0077693,0.0079668,0.0082118,0.0085126,0.0088775,0.0093177,0.0098501,0.010494,0.011271,0.012223,0.013393,0.014827,0.016573,0.018688,0.021065,0.023353,0.02514,0.025741,0.025766,0.02576;0.0068903,0.0069293,0.0070039,0.0071128,0.0072591,0.0074446,0.0076753,0.0079587,0.008303,0.0087195,0.0092225,0.0098328,0.010572,0.011476,0.012594,0.013981,0.015681,0.017769,0.020191,0.022618,0.024668,0.025516,0.025595,0.025593;0.0064698,0.0065049,0.006574,0.006676,0.0068138,0.006989,0.0072071,0.0074741,0.0078002,0.0081951,0.008673,0.0092517,0.009955,0.010818,0.011886,0.013225,0.014879,0.016928,0.019366,0.021908,0.024161,0.025263,0.025412,0.025411;0.0060997,0.0061318,0.0061962,0.006292,0.0064219,0.0065878,0.006794,0.0070472,0.0073565,0.0077323,0.0081866,0.0087375,0.0094085,0.010233,0.011257,0.012545,0.014154,0.01616,0.018596,0.021224,0.023646,0.024992,0.025219,0.025221;0.0057719,0.0058012,0.0058613,0.0059518,0.0060743,0.006232,0.0064275,0.0066679,0.0069624,0.0073201,0.0077535,0.0082795,0.0089208,0.0097104,0.010693,0.011932,0.013497,0.015458,0.017879,0.020565,0.023132,0.024704,0.025018,0.025025;0.0054794,0.0055061,0.0055623,0.0056477,0.0057645,0.0059136,0.0060997,0.0063293,0.0066096,0.0069515,0.0073655,0.0078687,0.0084832,0.0092404,0.010185,0.011379,0.012899,0.014818,0.017211,0.01994,0.022622,0.024403,0.02481,0.024823;0.0052168,0.0052407,0.005294,0.0053748,0.0054858,0.0056282,0.0058054,0.0060247,0.0062924,0.0066197,0.0070165,0.0074986,0.0080883,0.0088162,0.0097256,0.010878,0.012353,0.014228,0.016589,0.019344,0.022118,0.024093,0.024597,0.024612]  InterpMethod=Akima spline  RndMeth=Simplest
      settings: InputPortMap=u0,u1
  Lq_const : Constant  Value=Lq_t
  Mux : Mux  Inputs=[3, 2, 2, 3]
  Mux1 : Mux
  Mux2 : Mux  Inputs=[2, 1, 1, 1, 1]
  Mux3 : Mux  Inputs=2
  Mux4 : Mux  Inputs=2
  P : Constant  Value=P
  Psif(I_beta) : Lookup_n-D  BreakpointsForDimension1=[0,4,8,12,16,20,24,28,32,36,40,44,48,52,56,60,64,68,72,76]  BreakpointsForDimension2=[0,4,8,12,16,20,24,28,32,36,40,44,48,52,56,60,64,68,72,76,80,84,88,90]  Table=[0.098812,0.098812,0.098812,0.098812,0.098812,0.098812,0.098812,0.098812,0.098812,0.098812,0.098812,0.098812,0.098812,0.098812,0.098812,0.098812,0.098812,0.098812,0.098812,0.098812,0.098812,0.098812,0.098812,0.098812;0.10048,0.10244,0.104,0.10523,0.10621,0.107,0.10765,0.10817,0.10856,0.10888,0.10913,0.10932,0.10947,0.10958,0.10965,0.10969,0.10969,0.10971,0.10973,0.10973,0.10973,0.10972,0.10971,0.1097;0.10442,0.10813,0.11059,0.11225,0.1134,0.11418,0.11469,0.11497,0.11508,0.11505,0.11497,0.11478,0.11455,0.11425,0.11394,0.11362,0.1133,0.11298,0.11269,0.11247,0.11229,0.11217,0.1121,0.1121;0.10971,0.11589,0.11975,0.12184,0.12303,0.12353,0.12346,0.12308,0.12254,0.12191,0.12121,0.12046,0.11969,0.11884,0.11791,0.11705,0.11621,0.11543,0.11474,0.11417,0.11372,0.11342,0.11326,0.11324;0.11029,0.11747,0.12299,0.12605,0.12777,0.12873,0.12907,0.12908,0.12884,0.12842,0.12784,0.12689,0.12548,0.1239,0.12233,0.12077,0.11924,0.11782,0.11659,0.11556,0.11476,0.11423,0.11396,0.11393;0.11005,0.11803,0.12418,0.1279,0.13009,0.13139,0.13209,0.1323,0.13224,0.13209,0.13177,0.13124,0.13044,0.12915,0.12715,0.12485,0.12259,0.12041,0.11846,0.11687,0.11566,0.11485,0.11445,0.11439;0.10978,0.11858,0.12492,0.12891,0.13157,0.13321,0.13416,0.13462,0.13482,0.13483,0.13469,0.13436,0.13378,0.13288,0.13145,0.12917,0.12624,0.12328,0.12051,0.11822,0.1165,0.11537,0.11481,0.11474;0.10932,0.11886,0.12552,0.12974,0.13252,0.1344,0.13556,0.13626,0.13681,0.13714,0.13722,0.137,0.13656,0.13585,0.13471,0.13287,0.12998,0.12637,0.1228,0.11966,0.11734,0.11583,0.1151,0.115;0.10852,0.11876,0.12585,0.13038,0.13338,0.1355,0.1368,0.1377,0.13841,0.13893,0.1393,0.13937,0.13908,0.13845,0.13747,0.13588,0.13333,0.12955,0.12529,0.12125,0.11819,0.11624,0.1153,0.11519;0.10747,0.11845,0.12586,0.13067,0.13398,0.13623,0.13777,0.13896,0.13984,0.14054,0.14107,0.14137,0.14135,0.14089,0.13996,0.13851,0.1362,0.13254,0.12779,0.12296,0.119,0.11653,0.11537,0.11522;0.10635,0.118,0.12564,0.13073,0.13433,0.13678,0.1385,0.13993,0.14105,0.14195,0.14265,0.14314,0.14333,0.14311,0.14231,0.14092,0.13874,0.13521,0.13016,0.12474,0.11993,0.11686,0.11543,0.11524;0.10517,0.11745,0.12541,0.13063,0.13445,0.13713,0.13904,0.14067,0.14207,0.14317,0.1441,0.14476,0.14513,0.14511,0.14451,0.14318,0.14104,0.13763,0.13254,0.12656,0.12096,0.11718,0.11545,0.11523;0.10395,0.11682,0.12504,0.13049,0.13447,0.13734,0.13953,0.14139,0.14297,0.14431,0.14543,0.14626,0.14676,0.14689,0.14651,0.14529,0.14325,0.13995,0.13486,0.12838,0.12203,0.11753,0.11544,0.11519;0.10276,0.11613,0.12463,0.13031,0.13449,0.1375,0.13993,0.14203,0.14384,0.14536,0.14667,0.14768,0.1483,0.14859,0.14836,0.14735,0.14535,0.14212,0.13702,0.13016,0.12313,0.11787,0.11539,0.11509;0.10156,0.1154,0.12417,0.13005,0.13438,0.13766,0.14035,0.14264,0.14468,0.14641,0.14787,0.14904,0.14982,0.1502,0.15009,0.14928,0.14738,0.14419,0.13906,0.1319,0.12425,0.11823,0.11534,0.11499;0.10039,0.11469,0.12364,0.12971,0.13429,0.13787,0.14078,0.14323,0.14549,0.14744,0.14908,0.15039,0.15131,0.15178,0.15177,0.15112,0.14932,0.14616,0.14103,0.13362,0.12538,0.11863,0.11529,0.11488;0.099234,0.11395,0.1231,0.12941,0.13422,0.13808,0.14119,0.14387,0.1463,0.14848,0.15028,0.15174,0.15277,0.15335,0.15345,0.15289,0.15121,0.1481,0.14294,0.13532,0.12653,0.11904,0.11523,0.11476;0.098088,0.11321,0.12261,0.12916,0.1342,0.13832,0.14162,0.14454,0.14714,0.1495,0.15149,0.15309,0.15423,0.15493,0.15508,0.15462,0.15305,0.14998,0.14482,0.137,0.1277,0.11947,0.11519,0.11465;0.096962,0.11249,0.12213,0.12891,0.13424,0.13858,0.1421,0.14524,0.14802,0.15058,0.15273,0.15446,0.15571,0.15649,0.15674,0.15633,0.15488,0.15185,0.14667,0.13866,0.12887,0.11989,0.11508,0.11448;0.095857,0.11178,0.12171,0.12869,0.13431,0.13891,0.14261,0.14597,0.14896,0.1517,0.15401,0.15587,0.15722,0.15808,0.15838,0.15803,0.1567,0.15371,0.14849,0.14029,0.12999,0.12027,0.11494,0.11428]  InterpMethod=Akima spline  RndMeth=Simplest
      settings: InputPortMap=u0,u1
  R : Constant  Value=Rs
  Selector : Selector  InputPortWidth=3  IndexOptions=Index vector (dialog)  Indices=[1 2]  OutputSizes=1
  Subsystem : Subsystem
  Subsystem1 : Subsystem
  Subsystem2 : Subsystem
  Wb : Constant  Value=Flux_t
  abc2qd : Subsystem
  flux_const : Constant  Value=Flux_t
  phi d accurate1 : Lookup_n-D  Commented=on  BreakpointsForDimension1="[0     3     6     9    12    15    18    21    24    27    30]"  BreakpointsForDimension2="[0     3     6     9    12    15    18    21    24    27    30]"  Table=|  RndMeth=Simplest
      | [0.0227	0.0222	0.021833333	0.0215	0.021233333	0.021	0.0208	0.020633333	0.0205	0.020366667	0.0202;
      | 0.0227	0.0222	0.021833333	0.0215	0.021233333	0.021	0.0208	0.020633333	0.0205	0.020366667	0.0202;
      | 0.02265	0.022283333	0.021916667	0.0216	0.021333333	0.021083333	0.020883333	0.020683333	0.0205	0.020283333	0.02005;
      | 0.022433333	0.022144444	0.021822222	0.021522222	0.021244444	0.020977778	0.020711111	0.020433333	0.020144444	0.019844444	0.019511111;
      | 0.021375	0.021183333	0.020916667	0.020641667	0.020358333	0.020066667	0.019758333	0.019425	0.019075	0.018708333	0.018316667;
      | 0.0192	0.019106667	0.01894	0.01874	0.01852	0.018273333	0.018006667	0.01772	0.017413333	0.017086667	0.01674;
      | 0.0171	0.017055556	0.01695	0.016811111	0.01665	0.016461111	0.016255556	0.016033333	0.015788889	0.015522222	0.015244444;
      | 0.01537619	0.015347619	0.015280952	0.015180952	0.015061905	0.014919048	0.014757143	0.014580952	0.014385714	0.01417619	0.013957143;
      | 0.013979167	0.0139625	0.0139125	0.013841667	0.013745833	0.0136375	0.013508333	0.013366667	0.0132125	0.013041667	0.0128625;
      | 0.012833333	0.012818519	0.012785185	0.01272963	0.012659259	0.01257037	0.012466667	0.012351852	0.012225926	0.012085185	0.011937037;
      | 0.011876667	0.011866667	0.01184	0.011796667	0.01174	0.01167	0.011586667	0.01149	0.011386667	0.01127	0.011146667;]
      settings: InputPortMap=u0,u1
  phi q accurate1 : Lookup_n-D  Commented=on  BreakpointsForDimension1="[0     3     6     9    12    15    18    21    24    27    30]"  BreakpointsForDimension2="[0     3     6     9    12    15    18    21    24    27    30]"  Table=|  RndMeth=Simplest
      | [0.010733333	0.010733333	0.00825	0.007344444	0.006841667	0.00652	0.0063	0.006133333	0.006004167	0.0059	0.005816667;
      | 0.0105	0.0105	0.008183333	0.007288889	0.006808333	0.0065	0.006283333	0.00612381	0.005995833	0.005896296	0.005806667;
      | 0.009833333	0.009833333	0.007916667	0.007144444	0.006716667	0.006433333	0.006238889	0.006085714	0.005966667	0.005866667	0.005776667;
      | 0.008966667	0.008966667	0.007516667	0.0069	0.00655	0.006313333	0.006138889	0.006	0.0058875	0.005788889	0.0057;
      | 0.0079	0.0079	0.007016667	0.006566667	0.0063	0.006113333	0.005966667	0.005842857	0.005741667	0.005648148	0.005563333;
      | 0.007033333	0.007033333	0.0065	0.0062	0.006	0.005853333	0.005738889	0.005638095	0.00555	0.005466667	0.005393333;
      | 0.006433333	0.006433333	0.006083333	0.005877778	0.005725	0.005606667	0.005511111	0.005428571	0.005354167	0.005285185	0.005216667;
      | 0.006033333	0.006033333	0.00575	0.005588889	0.005475	0.005386667	0.005305556	0.005233333	0.005170833	0.005111111	0.00505;
      | 0.0057	0.0057	0.005483333	0.005355556	0.005258333	0.005186667	0.005116667	0.005057143	0.005	0.004948148	0.004896667;
      | 0.005433333	0.005433333	0.005266667	0.005144444	0.005066667	0.005	0.004944444	0.004895238	0.004845833	0.0048	0.004753333;
      | 0.005233333	0.005233333	0.005083333	0.004966667	0.004891667	0.00484	0.004788889	0.004747619	0.004704167	0.004659259	0.00462;]
      settings: InputPortMap=u0,u1
  i : Outport  VectorParamsAs1DForOutWhenUnconnected=off
  m : Outport  Port=2  VectorParamsAs1DForOutWhenUnconnected=off
  Te : Outport  Port=3  VectorParamsAs1DForOutWhenUnconnected=off
  wires:
  V/1 -> abc2qd/1("Vab, Vbc")
  theta/1 -> Subsystem/1(theta), Subsystem1/1(theta), abc2qd/2(theta)
  Subsystem2/1(iq,id) -> Mux2/1, Mux/2, [iqid_con], Demux/1, Subsystem1/3(iq,id)
  Wb/1 -> [Wb]
  we/1 -> Subsystem2/2(we)
  abc2qd/1("s, c") -> Subsystem1/2(s,c)
  [Lq] -> Mux1/2
  P/1 -> [P]
  Mux1/1 -> Subsystem2/3(LdLqRWb)
  [Wb] -> Mux2/5
  Mux2/1 -> Fcn/1
  R/1 -> [R]
  [Ld] -> Mux1/1
  Fcn/1 -> Te/1
  abc2qd/2("vq, vd") -> [Vqd_model], Mux/3, Subsystem2/1(vq,vd)
  [Ld] -> Mux2/3
  Mux/1 -> m/1
  Subsystem1/1(is) -> Mux/1, Selector/1
  Selector/1 -> i/1
  [R] -> Mux1/3
  Subsystem/1(Hall) -> Mux/4
  [P] -> Mux2/2
  [Lq] -> Mux2/4
  [Wb] -> Mux1/4
  Demux/2 -> [id]
  Demux/1 -> [iq]
  Abs/1 -> phi q accurate1/2, phi d accurate1/2
  phi q accurate1/1 -> Goto/1
  Abs1/1 -> phi q accurate1/1, phi d accurate1/1
  phi d accurate1/1 -> Goto1/1
  From8/1 -> Abs1/1
  From9/1 -> Abs/1
  Ld(I_beta)/1 -> ?  "Ld_act"
  Mux3/1 -> [iqid_act]
  Constant10/1 -> [Rs_act]
  [iq] -> Mux3/1, Mux4/2
  Lq(I_beta)/1 -> ?  "Lq_act"
  Psif(I_beta)/1 -> [Psif_act]  "phif_act"
  [id] -> Mux3/2, Mux4/1
  Subsystem2/2(p_idiq_con) -> [p_idiq_con]
  Mux4/1 -> Fcn2/1, Fcn1/1
  Fcn1/1 -> Ld(I_beta)/1, Psif(I_beta)/1, Lq(I_beta)/1
  Fcn2/1 -> Psif(I_beta)/2, Lq(I_beta)/2, Ld(I_beta)/2
  Ld_const/1 -> [Ld]
  Lq_const/1 -> [Lq]
